simulink model "Ex1_ONOFF_Control_Step12"  (R2023b)
settings: Solver=VariableStepAuto  StartTime=0.0  StopTime=10.0  RelTol=1e-3
libraries: arduinolib x1, arduinosensorlib x1
settings Model: Creator=Alejandro  LastModifiedBy=Alejandro

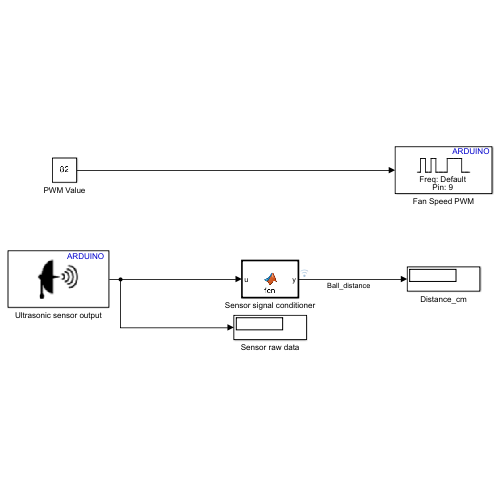
[thumbnail: Simulink's stored preview of the top-level diagram]
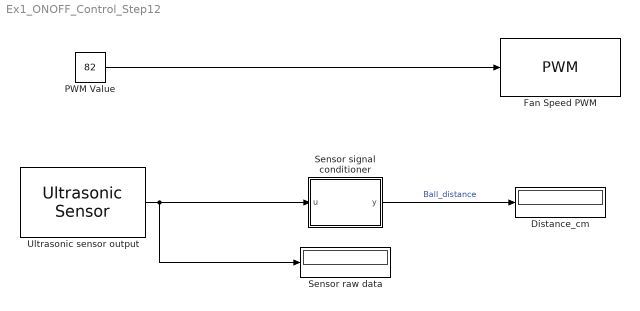
== system Ex1_ONOFF_Control_Step12 ==
  Distance_cm : Display
  Fan Speed PWM : arduinolib/PWM  pinNumber=9  frequencyType=Default  desiredFrequency=490.2  achievableFrequency=490.2
  PWM Value : Constant  Value=82
  Sensor raw data : Display
  Sensor signal conditioner : MATLAB Function  TreatAsAtomicUnit=on
  Ultrasonic sensor output : arduinosensorlib/Ultrasonic Sensor  NumSignalPins=2  TrigPin=12  EchoPin=11  SignalPin=3  SampleTime_=0.1  blockPlatform=ARDUINO
  wires:
  Sensor signal conditioner/1(y) -> Distance_cm/1  "Ball_distance"
  PWM Value/1 -> Fan Speed PWM/1
  Ultrasonic sensor output/1 -> Sensor signal conditioner/1(u), Sensor raw data/1

== matlab function Ex1_ONOFF_Control_Step12/Sensor signal conditioner ==
  data: u input; y output
function y = fcn(u)

MAX_DIST = 30;

y=MAX_DIST-(u*100);
